simulink model "RapidAccelFastRestart"  (R2025a)
settings: Solver=VariableStepAuto  StartTime=0.0  StopTime=10.0  RelTol=1e-3
values from neighbouring files (symbols this model uses):
  b = 1.0    [exFlexOp_dd.sldd]    (also in massSpringDamperDD.sldd = 100.0)
  F = 10.0    [massSpringDamperDD.sldd]
  k = 1000.0    [massSpringDamperDD.sldd]
  m = 10.0    [massSpringDamperDD.sldd]
settings Model: DataDictionary=massSpringDamperDD.sldd  SimulationMode=rapid-accelerator  Creator=grouleau  LastModifiedBy=grouleau

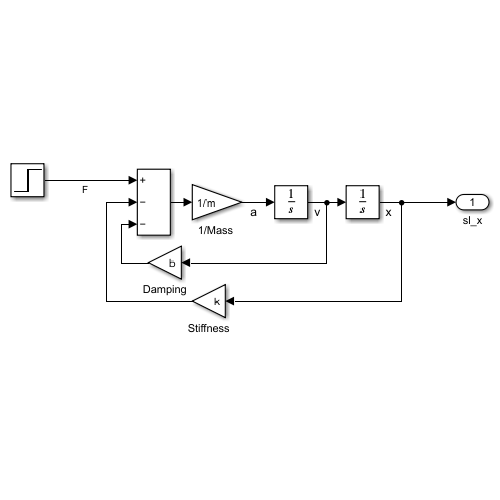
[thumbnail: Simulink's stored preview of the top-level diagram]
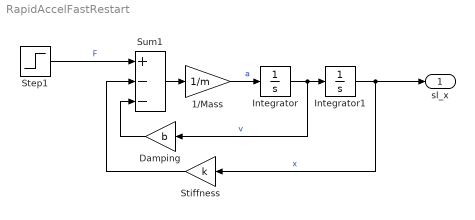
== system RapidAccelFastRestart ==
  "1/Mass " : Gain  Gain=1/m  SaturateOnIntegerOverflow=on  OutDataTypeStr=Inherit: Same as input  ParamDataTypeStr=Inherit: Same as input
  Damping : Gain  Gain=b  SaturateOnIntegerOverflow=on  OutDataTypeStr=Inherit: Same as input  ParamDataTypeStr=Inherit: Same as input
  Integrator : Integrator
  Integrator1 : Integrator
  Step1 : Step  After=F  SampleTime=0
  Stiffness : Gain  Gain=k  SaturateOnIntegerOverflow=on  OutDataTypeStr=Inherit: Same as input  ParamDataTypeStr=Inherit: Same as input
  Sum1 : Sum  Inputs=+--  InputSameDT=on  SaturateOnIntegerOverflow=on  OutDataTypeStr=Inherit: Same as first input
  sl_x : Outport
  wires:
  Stiffness/1 -> Sum1/2
  Damping/1 -> Sum1/3
  Step1/1 -> Sum1/1  "F"
  Integrator/1 -> Integrator1/1, Damping/1  "v"
  Integrator1/1 -> Stiffness/1, sl_x/1  "x"
  Sum1/1 -> "1/Mass "/1
  "1/Mass "/1 -> Integrator/1  "a"
